simulink model "platformController_harness"  (R2025b)
settings: Solver=FixedStepDiscrete  StartTime=0.0  StopTime=10  FixedStep=1/50  RelTol=1e-3
InitFcn:
  | plant_parameters;
  | fluid_constants;
undefined symbols (not defined in the file or in its folder): mass, mission_mode, platform_targets
libraries: simulink x7, slpidlib x3, matrix_library x1
settings Model: Creator=karadeli  LastModifiedBy=Kaan Kalkandelen
settings OptimizationCC: DefaultParameterBehavior=Inlined  UseDivisionForNetSlopeComputation=on  GainParamInheritBuiltInType=on  UseFloatMulNetSlope=on  PassReuseOutputArgsAs=Individual arguments  ZeroExternalMemoryAtStartup=off  ZeroInternalMemoryAtStartup=off  NoFixptDivByZeroProtection=on  EfficientFloat2IntCast=on  LifeSpan=1  OptimizeBlockOrder=speed  DifferentSizesBufferReuse=on  EfficientTunableParamExpr=on
settings DebuggingCC: ParameterTunabilityLossMsg=error
settings HardwareCC: ProdBitPerPointer=32.0  ProdBitPerSizeT=32.0  ProdBitPerPtrDiffT=32.0  ProdLargestAtomicInteger=Long  ProdLargestAtomicFloat=Double  ProdWordSize=32.0  ProdLongLongMode=on  ProdHWDeviceType=ARM Compatible->ARM Cortex-M
settings SFSimCC: MATLABDynamicMemAlloc=off
settings RTWCC: SystemTargetFile=ert.tlc  GenCodeOnly=on  TemplateMakefile=ert_default_tmf  TargetLang=C++  Description=Embedded Coder
settings CodeAppCC: ForceParamTrailComments=on  IgnoreCustomStorageClasses=off  OperatorAnnotations=on  SimulinkDataObjDesc=on  SFDataObjDesc=on  CustomSymbolStrGlobalVar=rt$N$M  CustomSymbolStrType=$N$M  CustomSymbolStrFcn=$N$M$F  CustomSymbolStrMacro=$N$M  InsertBlockDesc=on
settings ERTTargetCC: InlinedParameterPlacement=Hierarchical  RootIOFormat=Structure reference  ERTCustomFileTemplate=example_file_process.tlc  ERTFilePackagingFormat=CompactWithDataFile  TargetLangStandard=C++11 (ISO)  GenerateSampleERTMain=on  IncludeMdlTerminateFcn=off  CombineSignalStateStructs=on  SupportAbsoluteTime=off  CodeInterfacePackaging=C++ class  SubcomponentCodeInterfacePackaging=C++ class  SupportNonFinite=off  SupportComplex=off  SupportNonInlinedSFcns=on

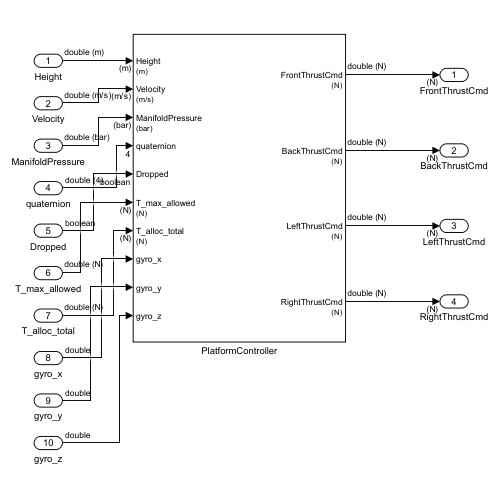
[thumbnail: Simulink's stored preview of the top-level diagram]
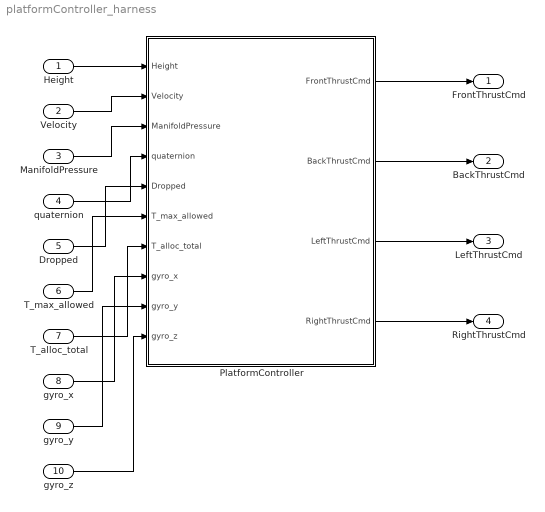
== system platformController_harness ==
  Height : Inport  Unit=m
  Velocity : Inport  Port=2  Unit=m/s
  ManifoldPressure : Inport  Port=3  Unit=bar
  quaternion : Inport  Port=4  PortDimensions=4
  Dropped : Inport  Port=5  OutDataTypeStr=boolean
  T_max_allowed : Inport  Port=6  Unit=N
  T_alloc_total : Inport  Port=7  Unit=N
  gyro_x : Inport  Port=8
  gyro_y : Inport  Port=9
  gyro_z : Inport  Port=10
  PlatformController : Subsystem
  FrontThrustCmd : Outport  Unit=N
  BackThrustCmd : Outport  Port=2  Unit=N
  LeftThrustCmd : Outport  Port=3  Unit=N
  RightThrustCmd : Outport  Port=4  Unit=N
  wires:
  T_max_allowed/1 -> PlatformController/6(T_max_allowed)
  T_alloc_total/1 -> PlatformController/7(T_alloc_total)
  Height/1 -> PlatformController/1(Height)
  Velocity/1 -> PlatformController/2(Velocity)
  quaternion/1 -> PlatformController/4(quaternion)
  ManifoldPressure/1 -> PlatformController/3(ManifoldPressure)
  Dropped/1 -> PlatformController/5(Dropped)
  PlatformController/1(FrontThrustCmd) -> FrontThrustCmd/1
  PlatformController/2(BackThrustCmd) -> BackThrustCmd/1
  PlatformController/3(LeftThrustCmd) -> LeftThrustCmd/1
  PlatformController/4(RightThrustCmd) -> RightThrustCmd/1
  gyro_x/1 -> PlatformController/8(gyro_x)
  gyro_y/1 -> PlatformController/9(gyro_y)
  gyro_z/1 -> PlatformController/10(gyro_z)

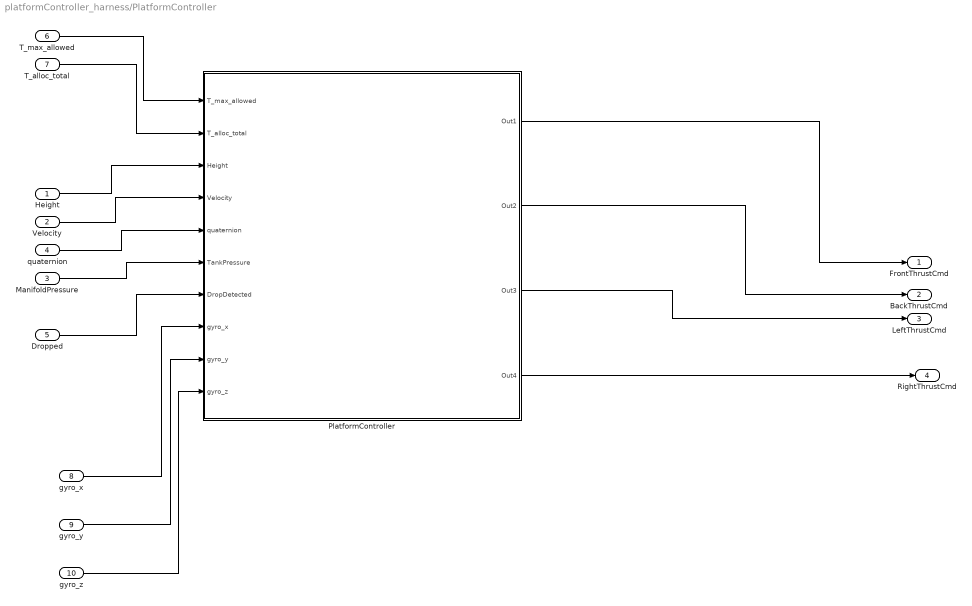
== system platformController_harness/PlatformController ==
  Height : Inport  Unit=m
  Velocity : Inport  Port=2  Unit=m/s
  ManifoldPressure : Inport  Port=3  Unit=bar
  quaternion : Inport  Port=4  PortDimensions=4
  Dropped : Inport  Port=5  OutDataTypeStr=boolean
  T_max_allowed : Inport  Port=6  Unit=N
  T_alloc_total : Inport  Port=7  Unit=N
  gyro_x : Inport  Port=8
  gyro_y : Inport  Port=9
  gyro_z : Inport  Port=10
  PlatformController : Subsystem
  FrontThrustCmd : Outport  Unit=N
  BackThrustCmd : Outport  Port=2  Unit=N
  LeftThrustCmd : Outport  Port=3  Unit=N
  RightThrustCmd : Outport  Port=4  Unit=N
  wires:
  T_max_allowed/1 -> PlatformController/1(T_max_allowed)
  T_alloc_total/1 -> PlatformController/2(T_alloc_total)
  Height/1 -> PlatformController/3(Height)
  Velocity/1 -> PlatformController/4(Velocity)
  quaternion/1 -> PlatformController/5(quaternion)
  ManifoldPressure/1 -> PlatformController/6(TankPressure)
  Dropped/1 -> PlatformController/7(DropDetected)
  gyro_x/1 -> PlatformController/8(gyro_x)
  gyro_y/1 -> PlatformController/9(gyro_y)
  gyro_z/1 -> PlatformController/10(gyro_z)
  PlatformController/1(Out1) -> FrontThrustCmd/1
  PlatformController/2(Out2) -> BackThrustCmd/1
  PlatformController/3(Out3) -> LeftThrustCmd/1
  PlatformController/4(Out4) -> RightThrustCmd/1

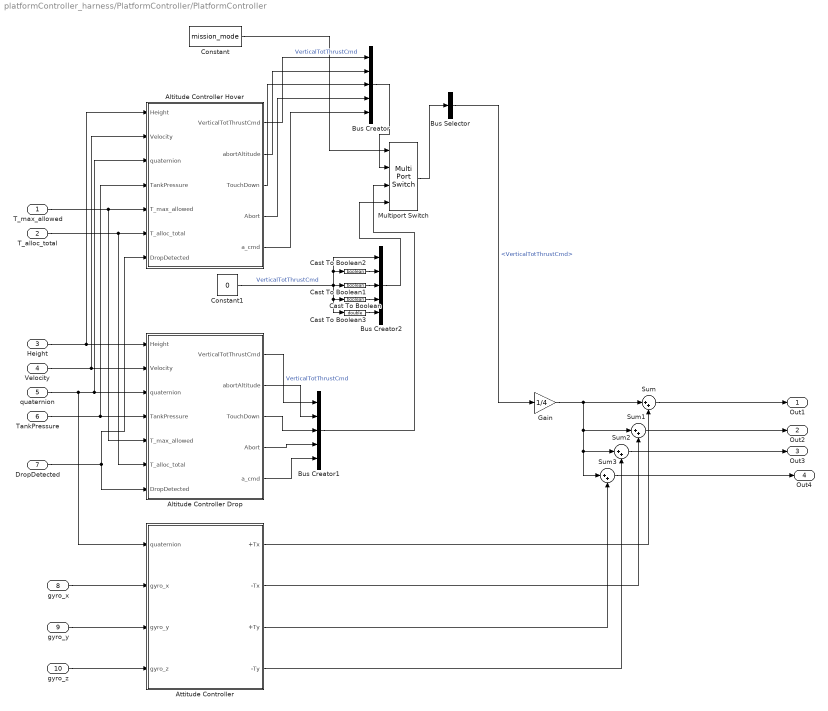
== system platformController_harness/PlatformController/PlatformController ==
  T_max_allowed : Inport
  T_alloc_total : Inport  Port=2
  Height : Inport  Port=3
  Velocity : Inport  Port=4
  quaternion : Inport  Port=5
  TankPressure : Inport  Port=6
  DropDetected : Inport  Port=7
  gyro_x : Inport  Port=8
  gyro_y : Inport  Port=9
  gyro_z : Inport  Port=10
  Altitude Controller Drop : Subsystem
  Altitude Controller Hover : Subsystem
  Attitude Controller : Subsystem
  Bus Creator : BusCreator  Inputs=5
  Bus Creator1 : BusCreator  Inputs=5
  Bus Creator2 : BusCreator  Inputs=5
  Bus Selector : BusSelector  OutputSignals=VerticalTotThrustCmd
  Cast To Boolean : DataTypeConversion  OutDataTypeStr=boolean  SaturateOnIntegerOverflow=off  RndMeth=Floor
  Cast To Boolean1 : DataTypeConversion  OutDataTypeStr=boolean  SaturateOnIntegerOverflow=off  RndMeth=Floor
  Cast To Boolean2 : DataTypeConversion  OutDataTypeStr=boolean  SaturateOnIntegerOverflow=off  RndMeth=Floor
  Cast To Boolean3 : DataTypeConversion  OutDataTypeStr=double  SaturateOnIntegerOverflow=off  RndMeth=Floor
  Constant : Constant  Value=mission_mode  OutDataTypeStr=Enum: mission_modes
  Constant1 : Constant  Value=0
  Gain : Gain  Gain=1/4
  Multiport Switch : MultiPortSwitch  DataPortOrder=Specify indices  DataPortIndices={mission_modes.HOVER, mission_modes.DROP}  DataPortForDefault=Additional data port  SaturateOnIntegerOverflow=off  InputSameDT=off
  Sum{,1..3} (4 alike) : Sum  Inputs=|++
  Out1 : Outport
  Out2 : Outport  Port=2
  Out3 : Outport  Port=3
  Out4 : Outport  Port=4
  wires:
  Cast To Boolean1/1 -> Bus Creator2/3
  T_alloc_total/1 -> Altitude Controller Drop/6(T_alloc_total), Altitude Controller Hover/6(T_alloc_total)
  Sum2/1 -> Out3/1
  T_max_allowed/1 -> Altitude Controller Drop/5(T_max_allowed), Altitude Controller Hover/5(T_max_allowed)
  Altitude Controller Hover/2(abortAltitude) -> Bus Creator/2
  Multiport Switch/1 -> Bus Selector/1
  Cast To Boolean/1 -> Bus Creator2/4
  Altitude Controller Hover/3(TouchDown) -> Bus Creator/3
  Attitude Controller/2(-Tx) -> Sum1/2
  quaternion/1 -> Attitude Controller/1(quaternion), Altitude Controller Drop/3(quaternion), Altitude Controller Hover/3(quaternion)
  Height/1 -> Altitude Controller Hover/1(Height), Altitude Controller Drop/1(Height)
  Velocity/1 -> Altitude Controller Hover/2(Velocity), Altitude Controller Drop/2(Velocity)
  Cast To Boolean3/1 -> Bus Creator2/5
  gyro_x/1 -> Attitude Controller/2(gyro_x)
  Altitude Controller Hover/1(VerticalTotThrustCmd) -> Bus Creator/1  "VerticalTotThrustCmd"
  Gain/1 -> Sum/1, Sum1/1, Sum3/1, Sum2/1
  Bus Selector/1 -> Gain/1  "<VerticalTotThrustCmd>"
  TankPressure/1 -> Altitude Controller Hover/4(TankPressure), Altitude Controller Drop/4(TankPressure)
  Altitude Controller Drop/4(Abort) -> Bus Creator1/4
  Constant1/1 -> Cast To Boolean1/1, Cast To Boolean/1, Cast To Boolean3/1, Cast To Boolean2/1, Bus Creator2/1  "VerticalTotThrustCmd"
  Attitude Controller/1(+Tx) -> Sum/2
  Attitude Controller/3(+Ty) -> Sum3/2
  Altitude Controller Drop/1(VerticalTotThrustCmd) -> Bus Creator1/1  "VerticalTotThrustCmd"
  Bus Creator/1 -> Multiport Switch/2
  Attitude Controller/4(-Ty) -> Sum2/2
  Bus Creator1/1 -> Multiport Switch/3
  Altitude Controller Hover/4(Abort) -> Bus Creator/4
  DropDetected/1 -> Altitude Controller Hover/7(DropDetected), Altitude Controller Drop/7(DropDetected)
  Altitude Controller Drop/3(TouchDown) -> Bus Creator1/3
  Sum/1 -> Out1/1
  Altitude Controller Drop/2(abortAltitude) -> Bus Creator1/2
  Altitude Controller Hover/5(a_cmd) -> Bus Creator/5
  Cast To Boolean2/1 -> Bus Creator2/2
  Constant/1 -> Multiport Switch/1
  Bus Creator2/1 -> Multiport Switch/4
  Altitude Controller Drop/5(a_cmd) -> Bus Creator1/5
  Sum1/1 -> Out2/1
  gyro_z/1 -> Attitude Controller/4(gyro_z)
  Sum3/1 -> Out4/1
  gyro_y/1 -> Attitude Controller/3(gyro_y)

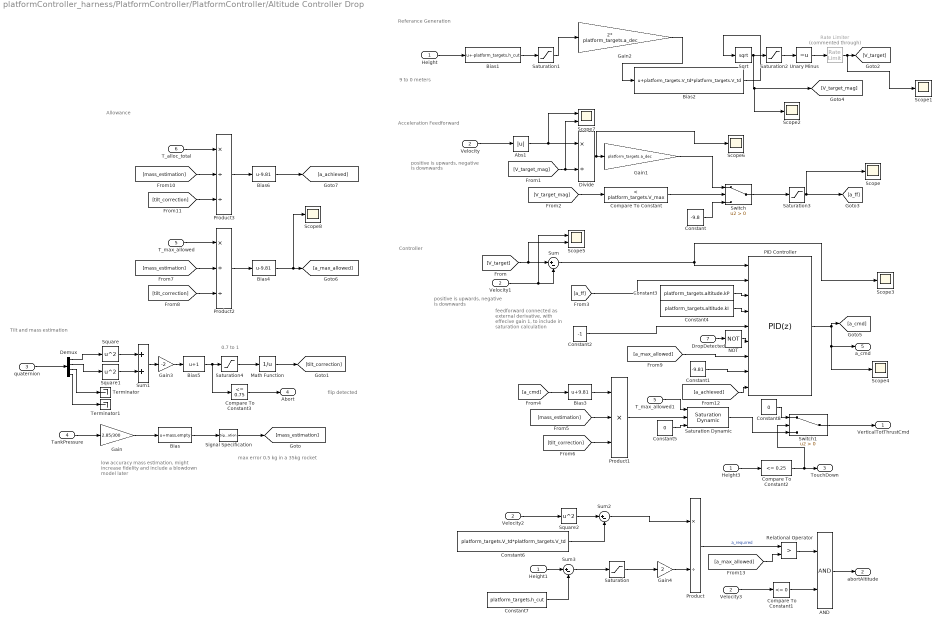
== system platformController_harness/PlatformController/PlatformController/Altitude Controller Drop ==
  note: flip detected
  note: max error 0.5 kg in a 35kg rocket
  note: 0.7 to 1
  note: Allowance
  note: Controller
  note: feedforward connected as external derivative, with effecive gain 1, to include in saturation calculation
  note: Tilt and mass estimation
  note: Acceleration Feedforward
  note: Referance Generation
  note: 9 to 0 meters
  note: low accuracy mass estimation, might increase fidelity and include a blowdown model later
  note: positive is upwards, negative is downwards
  note: positive is upwards, negative is downwards
  Height : Inport
  Velocity : Inport  Port=2
  quaternion : Inport  Port=3
  TankPressure : Inport  Port=4  Unit=bar
  T_max_allowed : Inport  Port=5  Unit=N
  T_alloc_total : Inport  Port=6
  DropDetected : Inport  Port=7
  AND : Logic  AllPortsSameDT=off  OutDataTypeStr=boolean
  Abs1 : Abs  SaturateOnIntegerOverflow=off
  Bias : Bias  Bias=mass.empty  SaturateOnIntegerOverflow=off
  Bias1 : Bias  Bias=-platform_targets.h_cut  SaturateOnIntegerOverflow=off
  Bias2 : Bias  Bias=platform_targets.V_td*platform_targets.V_td  SaturateOnIntegerOverflow=off
  Bias3 : Bias  Bias=9.81  SaturateOnIntegerOverflow=off
  Bias4 : Bias  Bias=-9.81  SaturateOnIntegerOverflow=off
  Bias5 : Bias  Bias=1  SaturateOnIntegerOverflow=off
  Bias6 : Bias  Bias=-9.81  SaturateOnIntegerOverflow=off
  Compare To Constant : simulink/Logic and Bit Operations/Compare To Constant  relop=<  const=platform_targets.V_max  OutDataTypeStr=boolean
  Compare To Constant1 : simulink/Logic and Bit Operations/Compare To Constant  relop=<=  const=0  OutDataTypeStr=boolean
  Compare To Constant2 : simulink/Logic and Bit Operations/Compare To Constant  relop=<=  const=0.25  OutDataTypeStr=boolean
  Compare To Constant3 : simulink/Logic and Bit Operations/Compare To Constant  relop=<=  const=0.75  OutDataTypeStr=boolean
  Constant : Constant  Value=-9.8
  Constant1 : Constant  Value=-9.81
  Constant2 : Constant  Value=-1
  Constant3 : Constant  Value=platform_targets.altitude.kP
  Constant4 : Constant  Value=platform_targets.altitude.kI
  Constant5 : Constant  Value=0
  Constant6 : Constant  Value=platform_targets.V_td*platform_targets.V_td
  Constant7 : Constant  Value=platform_targets.h_cut
  Constant8 : Constant  Value=0
  Demux : Demux
  Divide : Product  Inputs=*/
  Gain : Gain  Gain=2.85/300
  Gain1 : Gain  Gain=platform_targets.a_dec
  Gain2 : Gain  Gain=2* platform_targets.a_dec
  Gain3 : Gain  Gain=-2
  Gain4 : Gain  Gain=2
  Height1 : InportShadow
  Height3 : InportShadow
  Math Function : Math  Operator=reciprocal
  NOT : Logic  Operator=NOT  IconShape=distinctive  AllPortsSameDT=off  OutDataTypeStr=boolean
  PID Controller : slpidlib/PID Controller  Controller=PID  Form=Parallel  TimeDomain=Discrete-time  UseExternalTs=off  SampleTime=-1  IntegratorMethod=Forward Euler  FilterMethod=Forward Euler  ControllerParametersSource=external  P=1  I=1  UseKiTs=off  D=platform_targets.Ts  UseExternalDerivativeSource=on  N=100  UseFilter=off  TunerSelectOption=Frequency Response Based  InitialConditionSource=internal  InitialConditionForIntegrator=0  InitialConditionForFilter=0  DifferentiatorICPrevScaledInput=0  ExternalReset=rising  TrackingMode=on  Kt=1  LimitOutput=on  SatLimitsSource=external  UpperSaturationLimit=inf  LowerSaturationLimit=-inf  LinearizeAsGain=on  AntiWindupMode=clamping  Kb=1  LimitIntegrator=on  UpperIntegratorSaturationLimit=3  LowerIntegratorSaturationLimit=-3  POutMin=[]  POutMax=[]  IOutMin=[]  IOutMax=[]  DOutMin=[]  DOutMax=[]  NOutMin=[]  NOutMax=[]  SumOutMin=[]  SumOutMax=[]  SaturationOutMin=[]  SaturationOutMax=[]  PParamMin=[]  PParamMax=[]  IParamMin=[]  IParamMax=[]  DParamMin=[]  DParamMax=[]  NParamMin=[]  NParamMax=[]  KbParamMin=[]  KbParamMax=[]  KtParamMin=[]  KtParamMax=[]  KbOutMin=[]  KbOutMax=[]  KtOutMin=[]  KtOutMax=[]  IntegratorOutMin=[]  IntegratorOutMax=[]  FilterOutMin=[]  FilterOutMax=[]  SumI1OutMin=[]  SumI1OutMax=[]  SumI2OutMin=[]  SumI2OutMax=[]  SumI3OutMin=[]  SumI3OutMax=[]  SumI4OutMin=[]  SumI4OutMax=[]  SumDOutMin=[]  SumDOutMax=[]  DifferentiatorOutMin=[]  DifferentiatorOutMax=[]  FilterDiffOutCoefMin=[]  FilterDiffOutCoefMax=[]  ReciprocalOutMin=[]  ReciprocalOutMax=[]  SumDenOutMin=[]  SumDenOutMax=[]  SumNumOutMin=[]  SumNumOutMax=[]  DivideOutMin=[]  DivideOutMax=[]  UdiffTsProdOutMin=[]  UdiffTsProdOutMax=[]  NTsProdOutMin=[]  NTsProdOutMax=[]  UintegralTsProdOutMin=[]  UintegralTsProdOutMax=[]  UngainTsProdOutMin=[]  UngainTsProdOutMax=[]  ClampingZeroOutDataTypeStr=Inherit: Inherit via back propagation  ClampingZeroOutMin=[]  ClampingZeroOutMax=[]  FilterDenConstantOutDataTypeStr=Inherit: Inherit via back propagation  FilterDenConstantOutMin=[]  FilterDenConstantOutMax=[]  PCopyOutDataTypeStr=Inherit: Inherit via back propagation  PCopyOutMin=[]  PCopyOutMax=[]  NCopyOutDataTypeStr=Inherit: Inherit via back propagation  NCopyOutMin=[]  NCopyOutMax=[]  IntegratorContinuousStateAttributes=''  IntegratorStateMustResolveToSignalObject=off  IntegratorRTWStateStorageClass=Auto  FilterContinuousStateAttributes=''  FilterStateMustResolveToSignalObject=off  FilterRTWStateStorageClass=Auto  ParallelPVariant=ExternalParameters  IdealPVariant=Disabled  IVariant=ExternalParameters  DVariant=ExternalParameters  IntegratorVariant=Discrete  SatVariant=External  AWVariant=DiscClampingParallel  PCopyVariant=Disabled  TRVariant=Enabled  FdbkBlocksVariant=Forward  IdealPFdbkVariant=Disabled  SatFdbkVariant=Disabled  DerivativeFilterVariant=Passthrough  NVariant=Passthrough  NCopyVariant=Disabled_SignalSpec  FilterICVariant=Disabled  IntegratorICVariant=InternalICs  ExternalResetVariant=ExternalReset  TRSumVariant=TrackingMode  SumFdbkVariant=Disabled  SumVariant=Sum_PID  TsampFilterVariant=InternalTs  TsampNgainVariant=Passthrough  TsampIntegralVariant=Disabled_SignalSpec  ExternalSaturationOutDataTypeStr=Inherit: Same as second input  DerivativeSourceVariant=ExternalYdot  PreIntVariant=InternalPreInt
  Product : Product  Inputs=*/
  Product1 : Product  Inputs=3
  Product2 : Product  Inputs=*//
  Product3 : Product  Inputs=*//
  Rate Limiter : RateLimiter  Commented=through  RisingSlewLimit=1.5*platform_targets.a_dec  FallingSlewLimit=-1.5*platform_targets.a_dec  SampleTimeMode=inherited
  Relational Operator : RelationalOperator  Operator=>  OutDataTypeStr=boolean  RndMeth=Simplest  InputSameDT=off
  Saturation : Saturate  UpperLimit=0.1  LowerLimit=-inf
  Saturation Dynamic : simulink/Discontinuities/Saturation Dynamic  OutMin=[]  OutMax=[]  OutDataTypeStr=Inherit: Same as second input  OutDataType=fixdt(1, 16)  OutScaling=2^-10  DoSatur=off
  Saturation1 : Saturate  UpperLimit=inf  LowerLimit=0
  Saturation2 : Saturate  UpperLimit=platform_targets.V_max  LowerLimit=-inf
  Saturation3 : Saturate  UpperLimit=platform_targets.a_dec  LowerLimit=-inf
  Saturation4 : Saturate  UpperLimit=1  LowerLimit=0.7
  Scope{,1..4,6,8} (7 alike) : Scope
      Scope settings: ActiveDisplayYMinimum=-11.775  ActiveDisplayYMaximum=7.975
      Scope1 settings: ActiveDisplayYMinimum=-1  ActiveDisplayYMaximum=1  DataLoggingVariableName=ScopeData2
      Scope2 settings: ActiveDisplayYMinimum=-1.827770577815089  ActiveDisplayYMaximum=17.449935200335805  DataLoggingVariableName=ScopeData3
      Scope3 settings: ActiveDisplayYMinimum=-1  ActiveDisplayYMaximum=1  DataLoggingVariableName=ScopeData5
      Scope4 settings: ActiveDisplayYMinimum=-11.845500622839467  ActiveDisplayYMaximum=8.5095056055552  DataLoggingVariableName=ScopeData6
      Scope6 settings: ActiveDisplayYMinimum=-2.8207729738075158  ActiveDisplayYMaximum=25.386956764267644  DataLoggingVariableName=ScopeData10
      Scope8 settings: ActiveDisplayYMinimum=1.4571466713688759  ActiveDisplayYMaximum=13.020751190028783  DataLoggingVariableName=ScopeData17
  Scope5 : Scope  NumInputPorts=2
      settings: ActiveDisplayYMinimum=-11.352374051095602  ActiveDisplayYMaximum=1.2613748945661778  DataLoggingVariableName=ScopeData9
  Scope7 : Scope  NumInputPorts=2
      settings: ActiveDisplayYMinimum=-1  ActiveDisplayYMaximum=1  DataLoggingVariableName=ScopeData11
  Signal Specification : SignalSpecification  Unit=kg
  Sqrt : Sqrt
  Square : Math  Operator=square
  Square1 : Math  Operator=square
  Square2 : Math  Operator=square
  Sum : Sum  Inputs=|+-
  Sum1 : Sum  Inputs=2
  Sum2 : Sum  Inputs=|+-
  Sum3 : Sum  Inputs=|+-
  Switch : Switch  Criteria=u2 > Threshold  SaturateOnIntegerOverflow=off  InputSameDT=off
  Switch1 : Switch  Criteria=u2 > Threshold  SaturateOnIntegerOverflow=off  InputSameDT=off
  T_max_allowed1 : InportShadow  Port=5  Unit=N
  Terminator : Terminator
  Terminator1 : Terminator
  Unary Minus : UnaryMinus
  Velocity1 : InportShadow  Port=2
  Velocity2 : InportShadow  Port=2
  Velocity3 : InportShadow  Port=2
  VerticalTotThrustCmd : Outport  Unit=N
  abortAltitude : Outport  Port=2
  TouchDown : Outport  Port=3
  Abort : Outport  Port=4
  a_cmd : Outport  Port=5  Unit=m/s^2
  wires:
  Constant4/1 -> PID Controller/4
  Constant3/1 -> PID Controller/3
  [a_achieved] -> PID Controller/9
  Saturation3/1 -> [a_ff], Scope/1
  Compare To Constant3/1 -> Abort/1
  TankPressure/1 -> Gain/1
  Gain/1 -> Bias/1
  Bias/1 -> Signal Specification/1
  Signal Specification/1 -> [mass_estimation]
  Math Function/1 -> [tilt_correction]
  Height/1 -> Bias1/1
  Bias1/1 -> Saturation1/1
  Saturation1/1 -> Gain2/1
  Gain2/1 -> Bias2/1
  Bias2/1 -> Sqrt/1
  Unary Minus/1 -> Rate Limiter/1
  Saturation2/1 -> Unary Minus/1
  [V_target_mag] -> Compare To Constant/1
  Compare To Constant/1 -> Switch/2
  Constant/1 -> Switch/3
  Switch/1 -> Saturation3/1
  Velocity/1 -> Abs1/1
  Sqrt/1 -> [V_target_mag], Scope2/1, Saturation2/1
  [V_target_mag] -> Divide/2, Scope7/2
  Abs1/1 -> Divide/1, Scope7/1
  Divide/1 -> Gain1/1, Scope6/1
  Gain1/1 -> Switch/1
  [V_target] -> Sum/1, Scope5/2
  Velocity1/1 -> Sum/2, Scope5/1
  Constant1/1 -> PID Controller/8
  [a_max_allowed] -> PID Controller/7
  Sum/1 -> PID Controller/1, Scope3/1
  [a_ff] -> PID Controller/2
  Constant2/1 -> PID Controller/5
  PID Controller/1 -> a_cmd/1, Scope4/1, [a_cmd]
  [a_cmd] -> Bias3/1
  Bias3/1 -> Product1/1
  [mass_estimation] -> Product1/2
  [tilt_correction] -> Product1/3
  Product1/1 -> Saturation Dynamic/2
  Switch1/1 -> VerticalTotThrustCmd/1
  Constant5/1 -> Saturation Dynamic/3
  [tilt_correction] -> Product2/3
  [mass_estimation] -> Product2/2
  T_max_allowed/1 -> Product2/1
  Product2/1 -> Bias4/1
  Bias4/1 -> [a_max_allowed], Scope8/1
  T_max_allowed1/1 -> Saturation Dynamic/1
  Saturation4/1 -> Math Function/1
  quaternion/1 -> Demux/1
  Demux/1 -> Square/1
  Demux/2 -> Square1/1
  Demux/3 -> Terminator/1
  Square/1 -> Sum1/1
  Square1/1 -> Sum1/2
  Sum1/1 -> Gain3/1
  Gain3/1 -> Bias5/1
  Bias5/1 -> Compare To Constant3/1, Saturation4/1
  T_alloc_total/1 -> Product3/1
  [mass_estimation] -> Product3/2
  Product3/1 -> Bias6/1
  [tilt_correction] -> Product3/3
  Bias6/1 -> [a_achieved]
  Rate Limiter/1 -> [V_target], Scope1/1
  DropDetected/1 -> NOT/1
  NOT/1 -> PID Controller/6
  Velocity2/1 -> Square2/1
  Sum2/1 -> Product/1
  Square2/1 -> Sum2/1
  Constant6/1 -> Sum2/2
  Height1/1 -> Sum3/1
  Constant7/1 -> Sum3/2
  Sum3/1 -> Saturation/1
  Gain4/1 -> Product/2
  Saturation/1 -> Gain4/1
  Product/1 -> Relational Operator/1  "a_required"
  Relational Operator/1 -> AND/1
  [a_max_allowed] -> Relational Operator/2
  AND/1 -> abortAltitude/1
  Velocity3/1 -> Compare To Constant1/1
  Compare To Constant1/1 -> AND/2
  Demux/4 -> Terminator1/1
  Saturation Dynamic/1 -> Switch1/3
  Compare To Constant2/1 -> Switch1/2, TouchDown/1
  Height3/1 -> Compare To Constant2/1
  Constant8/1 -> Switch1/1

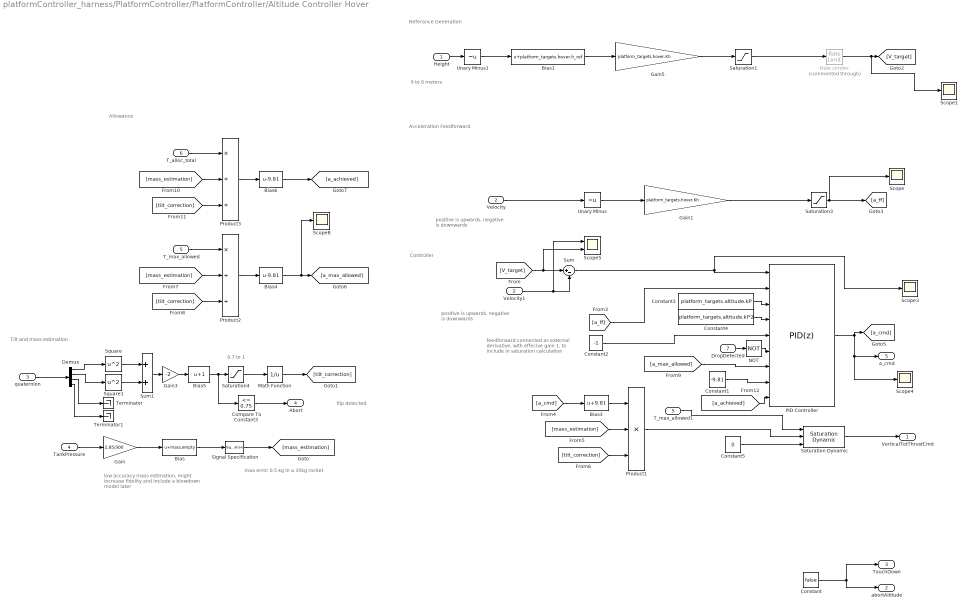
== system platformController_harness/PlatformController/PlatformController/Altitude Controller Hover ==
  note: positive is upwards, negative is downwards
  note: positive is upwards, negative is downwards
  note: low accuracy mass estimation, might increase fidelity and include a blowdown model later
  note: 9 to 0 meters
  note: Referance Generation
  note: Acceleration Feedforward
  note: Tilt and mass estimation
  note: feedforward connected as external derivative, with effecive gain 1, to include in saturation calculation
  note: Controller
  note: Allowance
  note: 0.7 to 1
  note: max error 0.5 kg in a 35kg rocket
  note: flip detected
  Height : Inport
  Velocity : Inport  Port=2
  quaternion : Inport  Port=3
  TankPressure : Inport  Port=4  Unit=bar
  T_max_allowed : Inport  Port=5  Unit=N
  T_alloc_total : Inport  Port=6
  DropDetected : Inport  Port=7
  Bias : Bias  Bias=mass.empty  SaturateOnIntegerOverflow=off
  Bias1 : Bias  Bias=platform_targets.hover.h_ref  SaturateOnIntegerOverflow=off
  Bias3 : Bias  Bias=9.81  SaturateOnIntegerOverflow=off
  Bias4 : Bias  Bias=-9.81  SaturateOnIntegerOverflow=off
  Bias5 : Bias  Bias=1  SaturateOnIntegerOverflow=off
  Bias6 : Bias  Bias=-9.81  SaturateOnIntegerOverflow=off
  Compare To Constant3 : simulink/Logic and Bit Operations/Compare To Constant  relop=<=  const=0.75  OutDataTypeStr=boolean
  Constant : Constant  Value=false
  Constant1 : Constant  Value=-9.81
  Constant2 : Constant  Value=-1
  Constant3 : Constant  Value=platform_targets.altitude.kP
  Constant4 : Constant  Value=platform_targets.altitude.kI*2
  Constant5 : Constant  Value=0
  Demux : Demux
  Gain : Gain  Gain=2.85/300
  Gain1 : Gain  Gain=platform_targets.hover.Kh
  Gain3 : Gain  Gain=-2
  Gain5 : Gain  Gain=platform_targets.hover.Kh
  Math Function : Math  Operator=reciprocal
  NOT : Logic  Operator=NOT  IconShape=distinctive  AllPortsSameDT=off  OutDataTypeStr=boolean
  PID Controller : slpidlib/PID Controller  Controller=PID  Form=Parallel  TimeDomain=Discrete-time  UseExternalTs=off  SampleTime=-1  IntegratorMethod=Forward Euler  FilterMethod=Forward Euler  ControllerParametersSource=external  P=1  I=1  UseKiTs=off  D=platform_targets.Ts  UseExternalDerivativeSource=on  N=100  UseFilter=off  TunerSelectOption=Frequency Response Based  InitialConditionSource=internal  InitialConditionForIntegrator=-9.81  InitialConditionForFilter=0  DifferentiatorICPrevScaledInput=0  ExternalReset=rising  TrackingMode=on  Kt=1  LimitOutput=on  SatLimitsSource=external  UpperSaturationLimit=inf  LowerSaturationLimit=-inf  LinearizeAsGain=on  AntiWindupMode=clamping  Kb=1  LimitIntegrator=on  UpperIntegratorSaturationLimit=3  LowerIntegratorSaturationLimit=-10  POutMin=[]  POutMax=[]  IOutMin=[]  IOutMax=[]  DOutMin=[]  DOutMax=[]  NOutMin=[]  NOutMax=[]  SumOutMin=[]  SumOutMax=[]  SaturationOutMin=[]  SaturationOutMax=[]  PParamMin=[]  PParamMax=[]  IParamMin=[]  IParamMax=[]  DParamMin=[]  DParamMax=[]  NParamMin=[]  NParamMax=[]  KbParamMin=[]  KbParamMax=[]  KtParamMin=[]  KtParamMax=[]  KbOutMin=[]  KbOutMax=[]  KtOutMin=[]  KtOutMax=[]  IntegratorOutMin=[]  IntegratorOutMax=[]  FilterOutMin=[]  FilterOutMax=[]  SumI1OutMin=[]  SumI1OutMax=[]  SumI2OutMin=[]  SumI2OutMax=[]  SumI3OutMin=[]  SumI3OutMax=[]  SumI4OutMin=[]  SumI4OutMax=[]  SumDOutMin=[]  SumDOutMax=[]  DifferentiatorOutMin=[]  DifferentiatorOutMax=[]  FilterDiffOutCoefMin=[]  FilterDiffOutCoefMax=[]  ReciprocalOutMin=[]  ReciprocalOutMax=[]  SumDenOutMin=[]  SumDenOutMax=[]  SumNumOutMin=[]  SumNumOutMax=[]  DivideOutMin=[]  DivideOutMax=[]  UdiffTsProdOutMin=[]  UdiffTsProdOutMax=[]  NTsProdOutMin=[]  NTsProdOutMax=[]  UintegralTsProdOutMin=[]  UintegralTsProdOutMax=[]  UngainTsProdOutMin=[]  UngainTsProdOutMax=[]  ClampingZeroOutDataTypeStr=Inherit: Inherit via back propagation  ClampingZeroOutMin=[]  ClampingZeroOutMax=[]  FilterDenConstantOutDataTypeStr=Inherit: Inherit via back propagation  FilterDenConstantOutMin=[]  FilterDenConstantOutMax=[]  PCopyOutDataTypeStr=Inherit: Inherit via back propagation  PCopyOutMin=[]  PCopyOutMax=[]  NCopyOutDataTypeStr=Inherit: Inherit via back propagation  NCopyOutMin=[]  NCopyOutMax=[]  IntegratorContinuousStateAttributes=''  IntegratorStateMustResolveToSignalObject=off  IntegratorRTWStateStorageClass=Auto  FilterContinuousStateAttributes=''  FilterStateMustResolveToSignalObject=off  FilterRTWStateStorageClass=Auto  ParallelPVariant=ExternalParameters  IdealPVariant=Disabled  IVariant=ExternalParameters  DVariant=ExternalParameters  IntegratorVariant=Discrete  SatVariant=External  AWVariant=DiscClampingParallel  PCopyVariant=Disabled  TRVariant=Enabled  FdbkBlocksVariant=Forward  IdealPFdbkVariant=Disabled  SatFdbkVariant=Disabled  DerivativeFilterVariant=Passthrough  NVariant=Passthrough  NCopyVariant=Disabled_SignalSpec  FilterICVariant=Disabled  IntegratorICVariant=InternalICs  ExternalResetVariant=ExternalReset  TRSumVariant=TrackingMode  SumFdbkVariant=Disabled  SumVariant=Sum_PID  TsampFilterVariant=InternalTs  TsampNgainVariant=Passthrough  TsampIntegralVariant=Disabled_SignalSpec  ExternalSaturationOutDataTypeStr=Inherit: Same as second input  DerivativeSourceVariant=ExternalYdot  PreIntVariant=InternalPreInt
  Product1 : Product  Inputs=3
  Product2 : Product  Inputs=*//
  Product3 : Product  Inputs=*//
  Rate Limiter : RateLimiter  Commented=through  RisingSlewLimit=1.5*platform_targets.a_dec  FallingSlewLimit=-1.5*platform_targets.a_dec  SampleTimeMode=inherited
  Saturation Dynamic : simulink/Discontinuities/Saturation Dynamic  OutMin=[]  OutMax=[]  OutDataTypeStr=Inherit: Same as second input  OutDataType=fixdt(1, 16)  OutScaling=2^-10  DoSatur=off
  Saturation1 : Saturate  UpperLimit=platform_targets.hover.v_sat(2)  LowerLimit=platform_targets.hover.v_sat(1)
  Saturation3 : Saturate  UpperLimit=platform_targets.a_dec_low  LowerLimit=-9.81
  Saturation4 : Saturate  UpperLimit=1  LowerLimit=0.7
  Scope{,1,3..4,8} (5 alike) : Scope
      Scope settings: ActiveDisplayYMinimum=-11.775  ActiveDisplayYMaximum=7.975
      Scope1 settings: ActiveDisplayYMinimum=-1  ActiveDisplayYMaximum=1  DataLoggingVariableName=ScopeData2
      Scope3 settings: ActiveDisplayYMinimum=-1  ActiveDisplayYMaximum=1  DataLoggingVariableName=ScopeData5
      Scope4 settings: ActiveDisplayYMinimum=-11.845500622839467  ActiveDisplayYMaximum=8.5095056055552  DataLoggingVariableName=ScopeData6
      Scope8 settings: ActiveDisplayYMinimum=1.4571466713688759  ActiveDisplayYMaximum=13.020751190028783  DataLoggingVariableName=ScopeData17
  Scope5 : Scope  NumInputPorts=2
      settings: ActiveDisplayYMinimum=-2.0131432669030809  ActiveDisplayYMaximum=3.1002766301241969  DataLoggingVariableName=ScopeData9
  Signal Specification : SignalSpecification  Unit=kg
  Square : Math  Operator=square
  Square1 : Math  Operator=square
  Sum : Sum  Inputs=|+-
  Sum1 : Sum  Inputs=2
  T_max_allowed1 : InportShadow  Port=5  Unit=N
  Terminator : Terminator
  Terminator1 : Terminator
  Unary Minus : UnaryMinus
  Unary Minus1 : UnaryMinus
  Velocity1 : InportShadow  Port=2
  VerticalTotThrustCmd : Outport  Unit=N
  abortAltitude : Outport  Port=2
  TouchDown : Outport  Port=3
  Abort : Outport  Port=4
  a_cmd : Outport  Port=5  Unit=m/s^2
  wires:
  Constant/1 -> abortAltitude/1, TouchDown/1
  Demux/4 -> Terminator1/1
  NOT/1 -> PID Controller/6
  DropDetected/1 -> NOT/1
  Rate Limiter/1 -> Scope1/1, [V_target]
  Bias6/1 -> [a_achieved]
  [tilt_correction] -> Product3/3
  Product3/1 -> Bias6/1
  [mass_estimation] -> Product3/2
  T_alloc_total/1 -> Product3/1
  Bias5/1 -> Saturation4/1, Compare To Constant3/1
  Gain3/1 -> Bias5/1
  Sum1/1 -> Gain3/1
  Square1/1 -> Sum1/2
  Square/1 -> Sum1/1
  Demux/3 -> Terminator/1
  Demux/2 -> Square1/1
  Demux/1 -> Square/1
  quaternion/1 -> Demux/1
  Saturation4/1 -> Math Function/1
  T_max_allowed1/1 -> Saturation Dynamic/1
  Bias4/1 -> Scope8/1, [a_max_allowed]
  Product2/1 -> Bias4/1
  T_max_allowed/1 -> Product2/1
  [mass_estimation] -> Product2/2
  [tilt_correction] -> Product2/3
  Constant5/1 -> Saturation Dynamic/3
  Saturation Dynamic/1 -> VerticalTotThrustCmd/1
  Product1/1 -> Saturation Dynamic/2
  [tilt_correction] -> Product1/3
  [mass_estimation] -> Product1/2
  Bias3/1 -> Product1/1
  [a_cmd] -> Bias3/1
  PID Controller/1 -> [a_cmd], Scope4/1, a_cmd/1
  Constant2/1 -> PID Controller/5
  [a_ff] -> PID Controller/2
  Sum/1 -> Scope3/1, PID Controller/1
  [a_max_allowed] -> PID Controller/7
  Constant1/1 -> PID Controller/8
  Velocity1/1 -> Scope5/1, Sum/2
  [V_target] -> Scope5/2, Sum/1
  Velocity/1 -> Unary Minus/1
  Gain1/1 -> Saturation3/1
  Saturation1/1 -> Rate Limiter/1
  Gain5/1 -> Saturation1/1
  Height/1 -> Unary Minus1/1
  Math Function/1 -> [tilt_correction]
  Signal Specification/1 -> [mass_estimation]
  Bias/1 -> Signal Specification/1
  Gain/1 -> Bias/1
  TankPressure/1 -> Gain/1
  Compare To Constant3/1 -> Abort/1
  Saturation3/1 -> Scope/1, [a_ff]
  [a_achieved] -> PID Controller/9
  Constant3/1 -> PID Controller/3
  Constant4/1 -> PID Controller/4
  Unary Minus1/1 -> Bias1/1
  Bias1/1 -> Gain5/1
  Unary Minus/1 -> Gain1/1

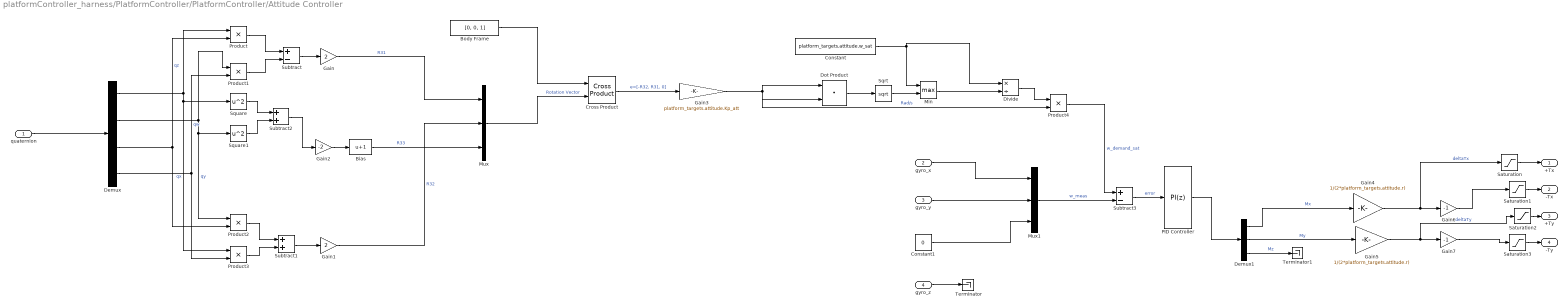
== system platformController_harness/PlatformController/PlatformController/Attitude Controller ==
  quaternion : Inport
  gyro_x : Inport  Port=2
  gyro_y : Inport  Port=3
  gyro_z : Inport  Port=4
  Bias : Bias  Bias=1  SaturateOnIntegerOverflow=off
  Body Frame : Constant  Value=[0, 0, 1]
  Constant : Constant  Value=platform_targets.attitude.w_sat
  Constant1 : Constant  Value=0
  Cross Product : matrix_library/Cross Product
  Demux : Demux
  Demux1 : Demux  Outputs=3
  Divide : Product  Inputs=*/
  Dot Product : DotProduct  OutDataTypeStr=Inherit: Inherit via internal rule
  Gain : Gain  Gain=2
  Gain1 : Gain  Gain=2
  Gain2 : Gain  Gain=-2
  Gain3 : Gain  Gain=platform_targets.attitude.Kp_att
  Gain4 : Gain  Gain=1/(2*platform_targets.attitude.r)
  Gain5 : Gain  Gain=1/(2*platform_targets.attitude.r)
  Gain6 : Gain  Gain=-1
  Gain7 : Gain  Gain=-1
  Min : MinMax  Function=max  Inputs=2
  Mux : Mux  Inputs=3
  Mux1 : Mux  Inputs=3
  PID Controller : slpidlib/PID Controller  Controller=PI  Form=Parallel  TimeDomain=Discrete-time  UseExternalTs=off  SampleTime=-1  IntegratorMethod=Forward Euler  FilterMethod=Forward Euler  ControllerParametersSource=internal  P=platform_targets.attitude.Kp_rate  I=platform_targets.attitude.Ki_rate  UseKiTs=off  D=0  UseExternalDerivativeSource=off  N=100  UseFilter=on  TunerSelectOption=Transfer Function Based (PID Tuner App)  InitialConditionSource=internal  InitialConditionForIntegrator=0  InitialConditionForFilter=0  DifferentiatorICPrevScaledInput=0  ExternalReset=none  TrackingMode=off  Kt=1  LimitOutput=off  SatLimitsSource=internal  UpperSaturationLimit=inf  LowerSaturationLimit=-inf  LinearizeAsGain=on  AntiWindupMode=none  Kb=1  LimitIntegrator=off  UpperIntegratorSaturationLimit=inf  LowerIntegratorSaturationLimit=-inf  POutMin=[]  POutMax=[]  IOutMin=[]  IOutMax=[]  DOutMin=[]  DOutMax=[]  NOutMin=[]  NOutMax=[]  SumOutMin=[]  SumOutMax=[]  SaturationOutMin=[]  SaturationOutMax=[]  PParamMin=[]  PParamMax=[]  IParamMin=[]  IParamMax=[]  DParamMin=[]  DParamMax=[]  NParamMin=[]  NParamMax=[]  KbParamMin=[]  KbParamMax=[]  KtParamMin=[]  KtParamMax=[]  KbOutMin=[]  KbOutMax=[]  KtOutMin=[]  KtOutMax=[]  IntegratorOutMin=[]  IntegratorOutMax=[]  FilterOutMin=[]  FilterOutMax=[]  SumI1OutMin=[]  SumI1OutMax=[]  SumI2OutMin=[]  SumI2OutMax=[]  SumI3OutMin=[]  SumI3OutMax=[]  SumI4OutMin=[]  SumI4OutMax=[]  SumDOutMin=[]  SumDOutMax=[]  DifferentiatorOutMin=[]  DifferentiatorOutMax=[]  FilterDiffOutCoefMin=[]  FilterDiffOutCoefMax=[]  ReciprocalOutMin=[]  ReciprocalOutMax=[]  SumDenOutMin=[]  SumDenOutMax=[]  SumNumOutMin=[]  SumNumOutMax=[]  DivideOutMin=[]  DivideOutMax=[]  UdiffTsProdOutMin=[]  UdiffTsProdOutMax=[]  NTsProdOutMin=[]  NTsProdOutMax=[]  UintegralTsProdOutMin=[]  UintegralTsProdOutMax=[]  UngainTsProdOutMin=[]  UngainTsProdOutMax=[]  ClampingZeroOutDataTypeStr=Inherit: Inherit via back propagation  ClampingZeroOutMin=[]  ClampingZeroOutMax=[]  FilterDenConstantOutDataTypeStr=Inherit: Inherit via back propagation  FilterDenConstantOutMin=[]  FilterDenConstantOutMax=[]  PCopyOutDataTypeStr=Inherit: Inherit via back propagation  PCopyOutMin=[]  PCopyOutMax=[]  NCopyOutDataTypeStr=Inherit: Inherit via back propagation  NCopyOutMin=[]  NCopyOutMax=[]  IntegratorContinuousStateAttributes=''  IntegratorStateMustResolveToSignalObject=off  IntegratorRTWStateStorageClass=Auto  FilterContinuousStateAttributes=''  FilterStateMustResolveToSignalObject=off  FilterRTWStateStorageClass=Auto  ParallelPVariant=InternalParameters  IdealPVariant=Disabled  IVariant=InternalParameters  DVariant=Disabled  IntegratorVariant=Discrete  SatVariant=Disabled  AWVariant=Passthrough  PCopyVariant=Disabled  TRVariant=Disabled  FdbkBlocksVariant=Forward  IdealPFdbkVariant=Disabled  SatFdbkVariant=Disabled  DerivativeFilterVariant=Disabled  NVariant=Disabled  NCopyVariant=Disabled_SignalSpec  FilterICVariant=Disabled  IntegratorICVariant=InternalICs  ExternalResetVariant=Disabled  TRSumVariant=Passthrough  SumFdbkVariant=Disabled  SumVariant=Sum_PI  TsampFilterVariant=InternalTs  TsampNgainVariant=Passthrough  TsampIntegralVariant=Disabled_SignalSpec  ExternalSaturationOutDataTypeStr=Inherit: Same as second input  DerivativeSourceVariant=Disabled  PreIntVariant=InternalPreInt
  Product{,1..4} (5 alike) : Product
  Saturation{,1..3} (4 alike) : Saturate  UpperLimit=272  LowerLimit=0
  Sqrt : Sqrt
  Square : Math  Operator=square
  Square1 : Math  Operator=square
  Subtract : Sum  Inputs=+-
  Subtract1 : Sum
  Subtract2 : Sum
  Subtract3 : Sum  Inputs=+-
  Terminator : Terminator
  Terminator1 : Terminator
  +Tx : Outport
  -Tx : Outport  Port=2
  +Ty : Outport  Port=3
  -Ty : Outport  Port=4
  wires:
  quaternion/1 -> Demux/1
  Cross Product/1 -> Gain3/1  "e=[-R32, R31, 0]"
  Bias/1 -> Mux/3  "R33"
  Mux/1 -> Cross Product/2  "Rotation Vector"
  Gain2/1 -> Bias/1
  Square/1 -> Subtract2/1
  Subtract1/1 -> Gain1/1
  Square1/1 -> Subtract2/2
  Subtract2/1 -> Gain2/1
  Product3/1 -> Subtract1/2
  Gain/1 -> Mux/1  "R31"
  Gain1/1 -> Mux/2  "R32"
  Product1/1 -> Subtract/2
  Product2/1 -> Subtract1/1
  Subtract/1 -> Gain/1
  Product/1 -> Subtract/1
  Demux/2 -> Square1/1, Product2/1, Product1/1  "qy"
  Demux/3 -> Product2/2, Product/2  "qz"
  Demux/1 -> Product3/1, Square/1, Product/1  "qx"
  Body Frame/1 -> Cross Product/1
  Demux/4 -> Product3/2, Product1/2  "qw"
  Gain3/1 -> Product4/2, Dot Product/2, Dot Product/1  "Rad/s"
  Dot Product/1 -> Sqrt/1
  Sqrt/1 -> Min/2
  Constant/1 -> Divide/1, Min/1
  Min/1 -> Divide/2
  Divide/1 -> Product4/1
  Product4/1 -> Subtract3/1  "w_demand_sat"
  gyro_x/1 -> Mux1/1
  gyro_y/1 -> Mux1/2
  gyro_z/1 -> Terminator/1
  Mux1/1 -> Subtract3/2  "w_meas"
  Constant1/1 -> Mux1/3
  Subtract3/1 -> PID Controller/1  "error"
  PID Controller/1 -> Demux1/1
  Demux1/1 -> Gain4/1  "Mx"
  Demux1/2 -> Gain5/1  "My"
  Demux1/3 -> Terminator1/1  "Mz"
  Gain4/1 -> Saturation/1, Gain6/1  "deltaTx"
  Gain6/1 -> Saturation1/1
  Gain7/1 -> Saturation3/1
  Gain5/1 -> Saturation2/1, Gain7/1  "deltaTy"
  Saturation/1 -> +Tx/1
  Saturation1/1 -> -Tx/1
  Saturation2/1 -> +Ty/1
  Saturation3/1 -> -Ty/1
